simulink library "halout"  (R2021b)
settings: Solver=VariableStepAuto  StartTime=0.0  StopTime=10.0  RelTol=1e-3
undefined symbols (not defined in the file): C_TASK_5MS_S, FALSE, KHAL_CAN1FDAPS3E2E_flg, KHAL_CAN1FDAPS3TxReq_flg, KHAL_CAN1FDVCU2E2E_flg, KHAL_CAN1FDVCU2TxReq_flg, KHAL_CAN1FDVCU3E2E_flg, KHAL_CAN1FDVCU3TxReq_flg, KHAL_CAN1TxReq_flg, KHAL_CAN2TxReq_flg, KHAL_CAN3FDVCU1TxReq_flg, KHAL_CAN3FDVCU2E2E_flg, KHAL_CAN3FDVCU2TxReq_flg, KHAL_CAN3TxReq_flg, KHAL_CAN4FDVCU1E2E_flg, KHAL_CAN4FDVCU1TxReq_flg, KHAL_CAN4TxReq_flg, KHAL_CAN5TxReq_flg, ONE_INT, TRUE, ZERO_INT
libraries: FVT_lib x383, simulink x179
(part 4 of 20)

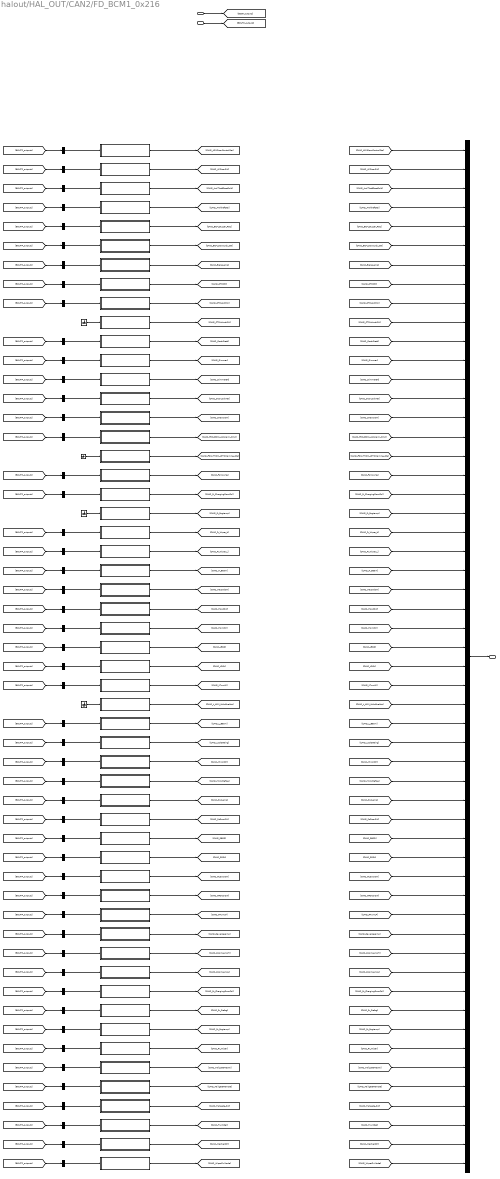
== system halout/HAL_OUT/CAN2/FD_BCM1_0x216 ==
  BSCP_outputs : Inport  OutDataTypeStr=Bus: BSCP_outputs
  BOUTP_outputs : Inport  Port=2  OutDataTypeStr=Bus: BOUTP_outputs
  APMDoorControlSta : Subsystem
  AllDoorSW : Subsystem
  AntiTheftSeatFold : Subsystem
  AntitheftSta : Subsystem
  BCMBuzzerReq : Subsystem
  BCMDoorLockSta : Subsystem
  BrakeLamp : Subsystem
  CTDCtrl : Subsystem
  CTDLockSW : Subsystem
  CTDUnlockSW : Subsystem
  CrashDetd : Subsystem
  Dimmer : Subsystem
  DimmerEN : Subsystem
  DoorLockIND : Subsystem
  DrDoorSW : Subsystem
  FDCBCMLockAlarmCmd : Subsystem
  FDCTHCMAPTCWarningSta : Subsystem
  FollowMe : Subsystem
  FrChargingDoorCtrl : Subsystem
  FrFogLamp : Subsystem
  FrWiperH : Subsystem
  FrWiperL : Subsystem
  Ground{,1..3} (4 alike) : Ground
  HBeam : Subsystem
  HazardSW : Subsystem
  HoodSW : Subsystem
  HornCtrl : Subsystem
  LAPMWdwEnable : Subsystem
  LBSD : Subsystem
  LBeam : Subsystem
  LDRL : Subsystem
  LTurnLP : Subsystem
  LockSetting : Subsystem
  MirrorCtrl : Subsystem
  MirrorDefog : Subsystem
  PosLamp : Subsystem
  PsDoorSW : Subsystem
  RBSD : Subsystem
  RDRL : Subsystem
  RLDoorSW : Subsystem
  RRDoorSW : Subsystem
  RTurnLP : Subsystem
  ReverseLamp : Subsystem
  RoomLampH : Subsystem
  RoomLampL : Subsystem
  RrChargingDoorCtrl : Subsystem
  RrDefog : Subsystem
  RrFogLamp : Subsystem
  RrWiper : Subsystem
  TailgateHDSW : Subsystem
  TailgateRemote : Subsystem
  TailgateSW : Subsystem
  TrunkRel : Subsystem
  WasherCtrl : Subsystem
  WiperFixMode : Subsystem
  bus_creator : BusCreator  Inputs=54  OutDataTypeStr=Bus: DT_CAN2_SG_FD_BCM1  NonVirtualBus=on
  bus_selector : BusSelector  OutputSignals=VOUTP_APMDoorControlSta_flg
  bus_selector1 : BusSelector  OutputSignals=VOUTP_AllDoorSW_flg
  bus_selector10 : BusSelector  OutputSignals=VOUTP_Dimmer_pct
  bus_selector11 : BusSelector  OutputSignals=VOUTP_DimmerEN_flg
  bus_selector12 : BusSelector  OutputSignals=VOUTP_DoorLockIND_flg
  bus_selector13 : BusSelector  OutputSignals=VOUTP_DrDoorSW_flg
  bus_selector14 : BusSelector  OutputSignals=VOUTP_LockAlarm_enum
  bus_selector16 : BusSelector  OutputSignals=VOUTP_FollowMe_flg
  bus_selector17 : BusSelector  OutputSignals=VOUTP_FrChargingDoorCtrl_enum
  bus_selector18 : BusSelector  OutputSignals=VOUTP_FrWiperH_flg
  bus_selector19 : BusSelector  OutputSignals=VOUTP_FrWiperL_flg
  bus_selector2 : BusSelector  OutputSignals=VOUTP_AntitheftSeatFlod_flg
  bus_selector20 : BusSelector  OutputSignals=VOUTP_HBeam_flg
  bus_selector21 : BusSelector  OutputSignals=VOUTP_HazardSW_flg
  bus_selector22 : BusSelector  OutputSignals=VOUTP_HoodSW_flg
  bus_selector23 : BusSelector  OutputSignals=VOUTP_HornCtrl_flg
  bus_selector24 : BusSelector  OutputSignals=VOUTP_LBSD_flg
  bus_selector25 : BusSelector  OutputSignals=VOUTP_LDRL_flg
  bus_selector26 : BusSelector  OutputSignals=VOUTP_LTurnLP_flg
  bus_selector27 : BusSelector  OutputSignals=VOUTP_LBeam_flg
  bus_selector28 : BusSelector  OutputSignals=VOUTP_LockSetting_flg
  bus_selector29 : BusSelector  OutputSignals=VOUTP_MirrorCtrl_enum
  bus_selector3 : BusSelector  OutputSignals=VOUTP_AntitheftSta_enum
  bus_selector30 : BusSelector  OutputSignals=VOUTP_MirrorDefog_flg
  bus_selector31 : BusSelector  OutputSignals=VOUTP_PosLamp_flg
  bus_selector32 : BusSelector  OutputSignals=VOUTP_PsDoorSW_flg
  bus_selector33 : BusSelector  OutputSignals=VOUTP_RBSD_flg
  bus_selector34 : BusSelector  OutputSignals=VOUTP_RDRL_flg
  bus_selector35 : BusSelector  OutputSignals=VOUTP_RLDoorSW_flg
  bus_selector36 : BusSelector  OutputSignals=VOUTP_RRDoorSW_flg
  bus_selector37 : BusSelector  OutputSignals=VOUTP_RTurnLP_flg
  bus_selector38 : BusSelector  OutputSignals=VOUTP_ReverseLamp_flg
  bus_selector39 : BusSelector  OutputSignals=VOUTP_RoomLampH_flg
  bus_selector4 : BusSelector  OutputSignals=VOUTP_BCMBuzzerReq_flg
  bus_selector40 : BusSelector  OutputSignals=VOUTP_RoomLampL_flg
  bus_selector41 : BusSelector  OutputSignals=VOUTP_RrChargingDoorCtrl_enum
  bus_selector42 : BusSelector  OutputSignals=VOUTP_RrDefog_flg
  bus_selector43 : BusSelector  OutputSignals=VOUTP_RrFogLamp_flg
  bus_selector44 : BusSelector  OutputSignals=VOUTP_RrWiper_flg
  bus_selector45 : BusSelector  OutputSignals=VOUTP_TailgateHDSW_flg
  bus_selector46 : BusSelector  OutputSignals=VOUTP_TailgateRemote_enum
  bus_selector47 : BusSelector  OutputSignals=VOUTP_TailgateSW_flg
  bus_selector48 : BusSelector  OutputSignals=VOUTP_TrunkRel_flg
  bus_selector49 : BusSelector  OutputSignals=VOUTP_WasherCtrl_enum
  bus_selector5 : BusSelector  OutputSignals=VOUTP_BCMDoorLockSta_flg
  bus_selector50 : BusSelector  OutputSignals=VOUTP_WiperFixMode_flg
  bus_selector6 : BusSelector  OutputSignals=VOUTP_BrakeLamp_flg
  bus_selector7 : BusSelector  OutputSignals=VOUTP_CTDCtrl_enum
  bus_selector8 : BusSelector  OutputSignals=VOUTP_CTDLockSW_flg
  bus_selector9 : BusSelector  OutputSignals=VOUTP_CrashDetd_flg
  FD_BCM1 : Outport
  wires:
  BSCP_outputs/1 -> [BSCP_outputs]
  BOUTP_outputs/1 -> [BOUTP_outputs]
  [CAN2_APMDoorControlSta] -> bus_creator/1  "CAN2_APMDoorControlSta"
  [CAN2_AllDoorSW] -> bus_creator/2  "CAN2_AllDoorSW"
  [CAN2_AntiTheftSeatFold] -> bus_creator/3  "CAN2_AntiTheftSeatFold"
  [CAN2_AntitheftSta] -> bus_creator/4  "CAN2_AntitheftSta"
  [CAN2_BCM_Buzzer_Req] -> bus_creator/5  "CAN2_BCM_Buzzer_Req"
  [CAN2_BCM_DoorLock_Sta] -> bus_creator/6  "CAN2_BCM_DoorLock_Sta"
  [CAN2_BrakeLamp] -> bus_creator/7  "CAN2_BrakeLamp"
  [CAN2_CTDCtrl] -> bus_creator/8  "CAN2_CTDCtrl"
  [CAN2_CTDLockSW] -> bus_creator/9  "CAN2_CTDLockSW"
  [CAN2_CTDUnlockSW] -> bus_creator/10  "CAN2_CTDUnlockSW"
  [CAN2_CrashDetd] -> bus_creator/11  "CAN2_CrashDetd"
  [CAN2_Dimmer] -> bus_creator/12  "CAN2_Dimmer"
  [CAN2_DimmerEN] -> bus_creator/13  "CAN2_DimmerEN"
  [CAN2_DoorLockIND] -> bus_creator/14  "CAN2_DoorLockIND"
  [CAN2_DrDoorSW] -> bus_creator/15  "CAN2_DrDoorSW"
  [CAN2_FDC_BCM_LockAlarm_Cmd] -> bus_creator/16  "CAN2_FDC_BCM_LockAlarm_Cmd"
  [CAN2_FDC_THCM_APTCWarning_Sta] -> bus_creator/17  "CAN2_FDC_THCM_APTCWarning_Sta"
  [CAN2_FollowMe] -> bus_creator/18  "CAN2_FollowMe"
  [CAN2_Fr_ChargingDoorCtrl] -> bus_creator/19  "CAN2_Fr_ChargingDoorCtrl"
  [CAN2_Fr_FogLamp] -> bus_creator/20  "CAN2_Fr_FogLamp"
  [CAN2_Fr_Wiper_H] -> bus_creator/21  "CAN2_Fr_Wiper_H"
  [CAN2_Fr_Wiper_L] -> bus_creator/22  "CAN2_Fr_Wiper_L"
  [CAN2_H_Beam] -> bus_creator/23  "CAN2_H_Beam"
  [CAN2_HazardSW] -> bus_creator/24  "CAN2_HazardSW"
  [CAN2_HoodSW] -> bus_creator/25  "CAN2_HoodSW"
  [CAN2_HornCtrl] -> bus_creator/26  "CAN2_HornCtrl"
  [CAN2_LBSD] -> bus_creator/27  "CAN2_LBSD"
  [CAN2_LDRL] -> bus_creator/28  "CAN2_LDRL"
  [CAN2_LTurnLP] -> bus_creator/29  "CAN2_LTurnLP"
  [CAN2_L_APM_WdwEnable] -> bus_creator/30  "CAN2_L_APM_WdwEnable"
  [CAN2_L_Beam] -> bus_creator/31  "CAN2_L_Beam"
  [CAN2_LockSetting] -> bus_creator/32  "CAN2_LockSetting"
  [CAN2_MirrorCtrl] -> bus_creator/33  "CAN2_MirrorCtrl"
  [CAN2_MirrorDefog] -> bus_creator/34  "CAN2_MirrorDefog"
  [CAN2_PosLamp] -> bus_creator/35  "CAN2_PosLamp"
  [CAN2_PsDoorSW] -> bus_creator/36  "CAN2_PsDoorSW"
  [CAN2_RBSD] -> bus_creator/37  "CAN2_RBSD"
  [CAN2_RDRL] -> bus_creator/38  "CAN2_RDRL"
  [CAN2_RLDoorSW] -> bus_creator/39  "CAN2_RLDoorSW"
  [CAN2_RRDoorSW] -> bus_creator/40  "CAN2_RRDoorSW"
  [CAN2_RTurnLP] -> bus_creator/41  "CAN2_RTurnLP"
  [CAN2_ReverseLamp] -> bus_creator/42  "CAN2_ReverseLamp"
  [CAN2_RoomLampH] -> bus_creator/43  "CAN2_RoomLampH"
  [CAN2_RoomLampL] -> bus_creator/44  "CAN2_RoomLampL"
  [CAN2_Rr_ChargingDoorCtrl] -> bus_creator/45  "CAN2_Rr_ChargingDoorCtrl"
  [CAN2_Rr_Defog] -> bus_creator/46  "CAN2_Rr_Defog"
  [CAN2_Rr_FogLamp] -> bus_creator/47  "CAN2_Rr_FogLamp"
  [CAN2_Rr_Wiper] -> bus_creator/48  "CAN2_Rr_Wiper"
  [CAN2_TailgateHDSW] -> bus_creator/49  "CAN2_TailgateHDSW"
  [CAN2_TailgateRemote] -> bus_creator/50  "CAN2_TailgateRemote"
  [CAN2_Tailgate_SW] -> bus_creator/51  "CAN2_Tailgate_SW"
  [CAN2_TrunkRel] -> bus_creator/52  "CAN2_TrunkRel"
  [CAN2_WasherCtrl] -> bus_creator/53  "CAN2_WasherCtrl"
  [CAN2_WiperFixMode] -> bus_creator/54  "CAN2_WiperFixMode"
  bus_creator/1 -> FD_BCM1/1
  APMDoorControlSta/1(CAN2_APMDoorControlSta) -> [CAN2_APMDoorControlSta]
  AllDoorSW/1(CAN2_AllDoorSW) -> [CAN2_AllDoorSW]
  AntiTheftSeatFold/1(CAN2_AntiTheftSeatFold) -> [CAN2_AntiTheftSeatFold]
  AntitheftSta/1(CAN2_AntitheftSta) -> [CAN2_AntitheftSta]
  BCMBuzzerReq/1(CAN2_BCM_Buzzer_Req) -> [CAN2_BCM_Buzzer_Req]
  BCMDoorLockSta/1(CAN2_BCM_DoorLock_Sta) -> [CAN2_BCM_DoorLock_Sta]
  BrakeLamp/1(CAN2_BrakeLamp) -> [CAN2_BrakeLamp]
  CTDCtrl/1(CAN2_CTDCtrl) -> [CAN2_CTDCtrl]
  CTDLockSW/1(CAN2_CTDLockSW) -> [CAN2_CTDLockSW]
  CTDUnlockSW/1(CAN2_CTDUnlockSW) -> [CAN2_CTDUnlockSW]
  CrashDetd/1(CAN2_CrashDetd) -> [CAN2_CrashDetd]
  Dimmer/1(CAN2_Dimmer) -> [CAN2_Dimmer]
  DimmerEN/1(CAN2_DimmerEN) -> [CAN2_DimmerEN]
  DoorLockIND/1(CAN2_DoorLockIND) -> [CAN2_DoorLockIND]
  DrDoorSW/1(CAN2_DrDoorSW) -> [CAN2_DrDoorSW]
  FDCBCMLockAlarmCmd/1(CAN2_FDC_BCM_LockAlarm_Cmd) -> [CAN2_FDC_BCM_LockAlarm_Cmd]
  FDCTHCMAPTCWarningSta/1(CAN2_FDC_THCM_APTCWarning_Sta) -> [CAN2_FDC_THCM_APTCWarning_Sta]
  FollowMe/1(CAN2_FollowMe) -> [CAN2_FollowMe]
  FrChargingDoorCtrl/1(CAN2_Fr_ChargingDoorCtrl) -> [CAN2_Fr_ChargingDoorCtrl]
  FrFogLamp/1(CAN2_Fr_FogLamp) -> [CAN2_Fr_FogLamp]
  FrWiperH/1(CAN2_Fr_Wiper_H) -> [CAN2_Fr_Wiper_H]
  FrWiperL/1(CAN2_Fr_Wiper_L) -> [CAN2_Fr_Wiper_L]
  HBeam/1(CAN2_H_Beam) -> [CAN2_H_Beam]
  HazardSW/1(CAN2_HazardSW) -> [CAN2_HazardSW]
  HoodSW/1(CAN2_HoodSW) -> [CAN2_HoodSW]
  HornCtrl/1(CAN2_HornCtrl) -> [CAN2_HornCtrl]
  LBSD/1(CAN2_LBSD) -> [CAN2_LBSD]
  LDRL/1(CAN2_LDRL) -> [CAN2_LDRL]
  LTurnLP/1(CAN2_LTurnLP) -> [CAN2_LTurnLP]
  LAPMWdwEnable/1(CAN2_L_APM_WdwEnable) -> [CAN2_L_APM_WdwEnable]
  LBeam/1(CAN2_L_Beam) -> [CAN2_L_Beam]
  LockSetting/1(CAN2_LockSetting) -> [CAN2_LockSetting]
  MirrorCtrl/1(CAN2_MirrorCtrl) -> [CAN2_MirrorCtrl]
  MirrorDefog/1(CAN2_MirrorDefog) -> [CAN2_MirrorDefog]
  PosLamp/1(CAN2_PosLamp) -> [CAN2_PosLamp]
  PsDoorSW/1(CAN2_PsDoorSW) -> [CAN2_PsDoorSW]
  RBSD/1(CAN2_RBSD) -> [CAN2_RBSD]
  RDRL/1(CAN2_RDRL) -> [CAN2_RDRL]
  RLDoorSW/1(CAN2_RLDoorSW) -> [CAN2_RLDoorSW]
  RRDoorSW/1(CAN2_RRDoorSW) -> [CAN2_RRDoorSW]
  RTurnLP/1(CAN2_RTurnLP) -> [CAN2_RTurnLP]
  ReverseLamp/1(CAN2_ReverseLamp) -> [CAN2_ReverseLamp]
  RoomLampH/1(CAN2_RoomLampH) -> [CAN2_RoomLampH]
  RoomLampL/1(CAN2_RoomLampL) -> [CAN2_RoomLampL]
  RrChargingDoorCtrl/1(CAN2_Rr_ChargingDoorCtrl) -> [CAN2_Rr_ChargingDoorCtrl]
  RrDefog/1(CAN2_Rr_Defog) -> [CAN2_Rr_Defog]
  RrFogLamp/1(CAN2_Rr_FogLamp) -> [CAN2_Rr_FogLamp]
  RrWiper/1(CAN2_Rr_Wiper) -> [CAN2_Rr_Wiper]
  TailgateHDSW/1(CAN2_TailgateHDSW) -> [CAN2_TailgateHDSW]
  TailgateRemote/1(CAN2_TailgateRemote) -> [CAN2_TailgateRemote]
  TailgateSW/1(CAN2_Tailgate_SW) -> [CAN2_Tailgate_SW]
  TrunkRel/1(CAN2_TrunkRel) -> [CAN2_TrunkRel]
  WasherCtrl/1(CAN2_WasherCtrl) -> [CAN2_WasherCtrl]
  WiperFixMode/1(CAN2_WiperFixMode) -> [CAN2_WiperFixMode]
  bus_selector/1 -> APMDoorControlSta/1(APMDoorControlSta)  "<VOUTP_APMDoorControlSta_flg>"
  [BOUTP_outputs] -> bus_selector/1
  bus_selector1/1 -> AllDoorSW/1(AllDoorSW)  "<VOUTP_AllDoorSW_flg>"
  [BOUTP_outputs] -> bus_selector1/1
  bus_selector2/1 -> AntiTheftSeatFold/1(AntiTheftSeatFold)  "<VOUTP_AntitheftSeatFlod_flg>"
  [BOUTP_outputs] -> bus_selector2/1
  bus_selector3/1 -> AntitheftSta/1(AntitheftSta)  "<VOUTP_AntitheftSta_enum>"
  [BOUTP_outputs] -> bus_selector3/1
  bus_selector4/1 -> BCMBuzzerReq/1(BCMBuzzerReq)  "<VOUTP_BCMBuzzerReq_flg>"
  [BOUTP_outputs] -> bus_selector4/1
  bus_selector5/1 -> BCMDoorLockSta/1(BCMDoorLockSta)  "<VOUTP_BCMDoorLockSta_flg>"
  [BOUTP_outputs] -> bus_selector5/1
  bus_selector6/1 -> BrakeLamp/1(BrakeLamp)  "<VOUTP_BrakeLamp_flg>"
  [BOUTP_outputs] -> bus_selector6/1
  bus_selector7/1 -> CTDCtrl/1(CTDCtrl)  "<VOUTP_CTDCtrl_enum>"
  [BOUTP_outputs] -> bus_selector7/1
  bus_selector8/1 -> CTDLockSW/1(CTDLockSW)  "<VOUTP_CTDLockSW_flg>"
  [BOUTP_outputs] -> bus_selector8/1
  Ground/1 -> CTDUnlockSW/1(CTDUnlockSW)
  bus_selector9/1 -> CrashDetd/1(CrashDetd)  "<VOUTP_CrashDetd_flg>"
  [BOUTP_outputs] -> bus_selector9/1
  bus_selector10/1 -> Dimmer/1(Dimmer)  "<VOUTP_Dimmer_pct>"
  [BOUTP_outputs] -> bus_selector10/1
  bus_selector11/1 -> DimmerEN/1(DimmerEN)  "<VOUTP_DimmerEN_flg>"
  [BOUTP_outputs] -> bus_selector11/1
  bus_selector12/1 -> DoorLockIND/1(DoorLockIND)  "<VOUTP_DoorLockIND_flg>"
  [BOUTP_outputs] -> bus_selector12/1
  bus_selector13/1 -> DrDoorSW/1(DrDoorSW)  "<VOUTP_DrDoorSW_flg>"
  [BOUTP_outputs] -> bus_selector13/1
  bus_selector14/1 -> FDCBCMLockAlarmCmd/1(FDCBCMLockAlarmCmd)  "<VOUTP_LockAlarm_enum>"
  [BOUTP_outputs] -> bus_selector14/1
  bus_selector16/1 -> FollowMe/1(FollowMe)  "<VOUTP_FollowMe_flg>"
  [BOUTP_outputs] -> bus_selector16/1
  bus_selector17/1 -> FrChargingDoorCtrl/1(FrChargingDoorCtrl)  "<VOUTP_FrChargingDoorCtrl_enum>"
  [BOUTP_outputs] -> bus_selector17/1
  Ground1/1 -> FrFogLamp/1(FrFogLamp)
  bus_selector18/1 -> FrWiperH/1(FrWiperH)  "<VOUTP_FrWiperH_flg>"
  [BOUTP_outputs] -> bus_selector18/1
  bus_selector19/1 -> FrWiperL/1(FrWiperL)  "<VOUTP_FrWiperL_flg>"
  [BOUTP_outputs] -> bus_selector19/1
  bus_selector20/1 -> HBeam/1(HBeam)  "<VOUTP_HBeam_flg>"
  [BOUTP_outputs] -> bus_selector20/1
  bus_selector21/1 -> HazardSW/1(HazardSW)  "<VOUTP_HazardSW_flg>"
  [BOUTP_outputs] -> bus_selector21/1
  bus_selector22/1 -> HoodSW/1(HoodSW)  "<VOUTP_HoodSW_flg>"
  [BOUTP_outputs] -> bus_selector22/1
  bus_selector23/1 -> HornCtrl/1(HornCtrl)  "<VOUTP_HornCtrl_flg>"
  [BOUTP_outputs] -> bus_selector23/1
  bus_selector24/1 -> LBSD/1(LBSD)  "<VOUTP_LBSD_flg>"
  [BOUTP_outputs] -> bus_selector24/1
  bus_selector25/1 -> LDRL/1(LDRL)  "<VOUTP_LDRL_flg>"
  [BOUTP_outputs] -> bus_selector25/1
  bus_selector26/1 -> LTurnLP/1(LTurnLP)  "<VOUTP_LTurnLP_flg>"
  [BOUTP_outputs] -> bus_selector26/1
  Ground2/1 -> LAPMWdwEnable/1(LAPMWdwEnable)
  bus_selector27/1 -> LBeam/1(LBeam)  "<VOUTP_LBeam_flg>"
  [BOUTP_outputs] -> bus_selector27/1
  bus_selector28/1 -> LockSetting/1(LockSetting)  "<VOUTP_LockSetting_flg>"
  [BOUTP_outputs] -> bus_selector28/1
  bus_selector29/1 -> MirrorCtrl/1(MirrorCtrl)  "<VOUTP_MirrorCtrl_enum>"
  [BOUTP_outputs] -> bus_selector29/1
  bus_selector30/1 -> MirrorDefog/1(MirrorDefog)  "<VOUTP_MirrorDefog_flg>"
  [BOUTP_outputs] -> bus_selector30/1
  bus_selector31/1 -> PosLamp/1(PosLamp)  "<VOUTP_PosLamp_flg>"
  [BOUTP_outputs] -> bus_selector31/1
  bus_selector32/1 -> PsDoorSW/1(PsDoorSW)  "<VOUTP_PsDoorSW_flg>"
  [BOUTP_outputs] -> bus_selector32/1
  bus_selector33/1 -> RBSD/1(RBSD)  "<VOUTP_RBSD_flg>"
  [BOUTP_outputs] -> bus_selector33/1
  bus_selector34/1 -> RDRL/1(RDRL)  "<VOUTP_RDRL_flg>"
  [BOUTP_outputs] -> bus_selector34/1
  bus_selector35/1 -> RLDoorSW/1(RLDoorSW)  "<VOUTP_RLDoorSW_flg>"
  [BOUTP_outputs] -> bus_selector35/1
  bus_selector36/1 -> RRDoorSW/1(RRDoorSW)  "<VOUTP_RRDoorSW_flg>"
  [BOUTP_outputs] -> bus_selector36/1
  bus_selector37/1 -> RTurnLP/1(RTurnLP)  "<VOUTP_RTurnLP_flg>"
  [BOUTP_outputs] -> bus_selector37/1
  bus_selector38/1 -> ReverseLamp/1(ReverseLamp)  "<VOUTP_ReverseLamp_flg>"
  [BOUTP_outputs] -> bus_selector38/1
  bus_selector39/1 -> RoomLampH/1(RoomLampH)  "<VOUTP_RoomLampH_flg>"
  [BOUTP_outputs] -> bus_selector39/1
  bus_selector40/1 -> RoomLampL/1(RoomLampL)  "<VOUTP_RoomLampL_flg>"
  [BOUTP_outputs] -> bus_selector40/1
  bus_selector41/1 -> RrChargingDoorCtrl/1(RrChargingDoorCtrl)  "<VOUTP_RrChargingDoorCtrl_enum>"
  [BOUTP_outputs] -> bus_selector41/1
  bus_selector42/1 -> RrDefog/1(RrDefog)  "<VOUTP_RrDefog_flg>"
  [BOUTP_outputs] -> bus_selector42/1
  bus_selector43/1 -> RrFogLamp/1(RrFogLamp)  "<VOUTP_RrFogLamp_flg>"
  [BOUTP_outputs] -> bus_selector43/1
  bus_selector44/1 -> RrWiper/1(RrWiper)  "<VOUTP_RrWiper_flg>"
  [BOUTP_outputs] -> bus_selector44/1
  bus_selector45/1 -> TailgateHDSW/1(TailgateHDSW)  "<VOUTP_TailgateHDSW_flg>"
  [BOUTP_outputs] -> bus_selector45/1
  bus_selector46/1 -> TailgateRemote/1(TailgateRemote)  "<VOUTP_TailgateRemote_enum>"
  [BOUTP_outputs] -> bus_selector46/1
  bus_selector47/1 -> TailgateSW/1(TailgateSW)  "<VOUTP_TailgateSW_flg>"
  [BOUTP_outputs] -> bus_selector47/1
  bus_selector48/1 -> TrunkRel/1(TrunkRel)  "<VOUTP_TrunkRel_flg>"
  [BOUTP_outputs] -> bus_selector48/1
  bus_selector49/1 -> WasherCtrl/1(WasherCtrl)  "<VOUTP_WasherCtrl_enum>"
  [BOUTP_outputs] -> bus_selector49/1
  bus_selector50/1 -> WiperFixMode/1(WiperFixMode)  "<VOUTP_WiperFixMode_flg>"
  [BOUTP_outputs] -> bus_selector50/1
  Ground3/1 -> FDCTHCMAPTCWarningSta/1(FDCTHCMAPTCWarningSta)

== system halout/HAL_OUT/CAN2/FD_BCM2_0x217 ==
  BSCP_outputs : Inport  OutDataTypeStr=Bus: BSCP_outputs
  BOUTP_outputs : Inport  Port=2  OutDataTypeStr=Bus: BOUTP_outputs
  AmbLightBreath1 : Subsystem
  AmbLightBreath2 : Subsystem
  AmbLightBreath3 : Subsystem
  AmbLightBrightness1 : Subsystem
  AmbLightBrightness2 : Subsystem
  AmbLightBrightness3 : Subsystem
  AmbLightColor1 : Subsystem
  AmbLightColor2 : Subsystem
  AmbLightColor3 : Subsystem
  LampPwr : Subsystem
  User1AmbLightColor : Subsystem
  User1DrAmbLightBrightness : Subsystem
  User1IPAmbLightBrightness : Subsystem
  User2AmbLightColor : Subsystem
  User2DrAmbLightBrightness : Subsystem
  User2IPAmbLightBrightness : Subsystem
  User3AmbLightColor : Subsystem
  User3DrAmbLightBrightness : Subsystem
  User3IPAmbLightBrightness : Subsystem
  User4AmbLightColor : Subsystem
  User4DrAmbLightBrightness : Subsystem
  User4IPAmbLightBrightness : Subsystem
  User5AmbLightColor : Subsystem
  User5DrAmbLightBrightness : Subsystem
  User5IPAmbLightBrightness : Subsystem
  User6AmbLightColor : Subsystem
  User6DrAmbLightBrightness : Subsystem
  User6IPAmbLightBrightness : Subsystem
  bus_creator : BusCreator  Inputs=28  OutDataTypeStr=Bus: DT_CAN2_SG_FD_BCM2  NonVirtualBus=on
  bus_selector : BusSelector  OutputSignals=VOUTP_AmbLightBreath1_flg
  bus_selector1 : BusSelector  OutputSignals=VOUTP_AmbLightBreath2_flg
  bus_selector10 : BusSelector  OutputSignals=VOUTP_User1AmbLightColor_enum
  bus_selector11 : BusSelector  OutputSignals=VOUTP_User1DrAmbLightBrightness_enum
  bus_selector12 : BusSelector  OutputSignals=VOUTP_User1IPAmbLightBrightness_enum
  bus_selector13 : BusSelector  OutputSignals=VOUTP_User2AmbLightColor_enum
  bus_selector14 : BusSelector  OutputSignals=VOUTP_User2DrAmbLightBrightness_enum
  bus_selector15 : BusSelector  OutputSignals=VOUTP_User2IPAmbLightBrightness_enum
  bus_selector16 : BusSelector  OutputSignals=VOUTP_User3AmbLightColor_enum
  bus_selector17 : BusSelector  OutputSignals=VOUTP_User3DrAmbLightBrightness_enum
  bus_selector18 : BusSelector  OutputSignals=VOUTP_User3IPAmbLightBrightness_enum
  bus_selector19 : BusSelector  OutputSignals=VOUTP_User4AmbLightColor_enum
  bus_selector2 : BusSelector  OutputSignals=VOUTP_AmbLightBreath3_flg
  bus_selector20 : BusSelector  OutputSignals=VOUTP_User4DrAmbLightBrightness_enum
  bus_selector21 : BusSelector  OutputSignals=VOUTP_User4IPAmbLightBrightness_enum
  bus_selector22 : BusSelector  OutputSignals=VOUTP_User5AmbLightColor_enum
  bus_selector23 : BusSelector  OutputSignals=VOUTP_User5DrAmbLightBrightness_enum
  bus_selector24 : BusSelector  OutputSignals=VOUTP_User5IPAmbLightBrightness_enum
  bus_selector25 : BusSelector  OutputSignals=VOUTP_User6AmbLightColor_enum
  bus_selector26 : BusSelector  OutputSignals=VOUTP_User6DrAmbLightBrightness_enum
  bus_selector27 : BusSelector  OutputSignals=VOUTP_User6IPAmbLightBrightness_enum
  bus_selector3 : BusSelector  OutputSignals=VOUTP_AmbLightBrightness1_enum
  bus_selector4 : BusSelector  OutputSignals=VOUTP_AmbLightBrightness2_enum
  bus_selector5 : BusSelector  OutputSignals=VOUTP_AmbLightBrightness3_enum
  bus_selector6 : BusSelector  OutputSignals=VOUTP_AmbLightColor1_enum
  bus_selector7 : BusSelector  OutputSignals=VOUTP_AmbLightColor2_enum
  bus_selector8 : BusSelector  OutputSignals=VOUTP_AmbLightColor3_enum
  bus_selector9 : BusSelector  OutputSignals=VOUTP_LampPwr_flg
  FD_BCM2 : Outport
  wires:
  BSCP_outputs/1 -> [BSCP_outputs]
  BOUTP_outputs/1 -> [BOUTP_outputs]
  [CAN2_AmbLightBreath1] -> bus_creator/1  "CAN2_AmbLightBreath1"
  [CAN2_AmbLightBreath2] -> bus_creator/2  "CAN2_AmbLightBreath2"
  [CAN2_AmbLightBreath3] -> bus_creator/3  "CAN2_AmbLightBreath3"
  [CAN2_AmbLightBrightness1] -> bus_creator/4  "CAN2_AmbLightBrightness1"
  [CAN2_AmbLightBrightness2] -> bus_creator/5  "CAN2_AmbLightBrightness2"
  [CAN2_AmbLightBrightness3] -> bus_creator/6  "CAN2_AmbLightBrightness3"
  [CAN2_AmbLightColor1] -> bus_creator/7  "CAN2_AmbLightColor1"
  [CAN2_AmbLightColor2] -> bus_creator/8  "CAN2_AmbLightColor2"
  [CAN2_AmbLightColor3] -> bus_creator/9  "CAN2_AmbLightColor3"
  [CAN2_LampPwr] -> bus_creator/10  "CAN2_LampPwr"
  [CAN2_User1AmbLightColor] -> bus_creator/11  "CAN2_User1AmbLightColor"
  [CAN2_User1DrAmbLightBrightness] -> bus_creator/12  "CAN2_User1DrAmbLightBrightness"
  [CAN2_User1IPAmbLightBrightness] -> bus_creator/13  "CAN2_User1IPAmbLightBrightness"
  [CAN2_User2AmbLightColor] -> bus_creator/14  "CAN2_User2AmbLightColor"
  [CAN2_User2DrAmbLightBrightness] -> bus_creator/15  "CAN2_User2DrAmbLightBrightness"
  [CAN2_User2IPAmbLightBrightness] -> bus_creator/16  "CAN2_User2IPAmbLightBrightness"
  [CAN2_User3AmbLightColor] -> bus_creator/17  "CAN2_User3AmbLightColor"
  [CAN2_User3DrAmbLightBrightness] -> bus_creator/18  "CAN2_User3DrAmbLightBrightness"
  [CAN2_User3IPAmbLightBrightness] -> bus_creator/19  "CAN2_User3IPAmbLightBrightness"
  [CAN2_User4AmbLightColor] -> bus_creator/20  "CAN2_User4AmbLightColor"
  [CAN2_User4DrAmbLightBrightness] -> bus_creator/21  "CAN2_User4DrAmbLightBrightness"
  [CAN2_User4IPAmbLightBrightness] -> bus_creator/22  "CAN2_User4IPAmbLightBrightness"
  [CAN2_User5AmbLightColor] -> bus_creator/23  "CAN2_User5AmbLightColor"
  [CAN2_User5DrAmbLightBrightness] -> bus_creator/24  "CAN2_User5DrAmbLightBrightness"
  [CAN2_User5IPAmbLightBrightness] -> bus_creator/25  "CAN2_User5IPAmbLightBrightness"
  [CAN2_User6AmbLightColor] -> bus_creator/26  "CAN2_User6AmbLightColor"
  [CAN2_User6DrAmbLightBrightness] -> bus_creator/27  "CAN2_User6DrAmbLightBrightness"
  [CAN2_User6IPAmbLightBrightness] -> bus_creator/28  "CAN2_User6IPAmbLightBrightness"
  bus_creator/1 -> FD_BCM2/1
  AmbLightBreath1/1(CAN2_AmbLightBreath1) -> [CAN2_AmbLightBreath1]
  AmbLightBreath2/1(CAN2_AmbLightBreath2) -> [CAN2_AmbLightBreath2]
  AmbLightBreath3/1(CAN2_AmbLightBreath3) -> [CAN2_AmbLightBreath3]
  AmbLightBrightness1/1(CAN2_AmbLightBrightness1) -> [CAN2_AmbLightBrightness1]
  AmbLightBrightness2/1(CAN2_AmbLightBrightness2) -> [CAN2_AmbLightBrightness2]
  AmbLightBrightness3/1(CAN2_AmbLightBrightness3) -> [CAN2_AmbLightBrightness3]
  AmbLightColor1/1(CAN2_AmbLightColor1) -> [CAN2_AmbLightColor1]
  AmbLightColor2/1(CAN2_AmbLightColor2) -> [CAN2_AmbLightColor2]
  AmbLightColor3/1(CAN2_AmbLightColor3) -> [CAN2_AmbLightColor3]
  LampPwr/1(CAN2_LampPwr) -> [CAN2_LampPwr]
  User1AmbLightColor/1(CAN2_User1AmbLightColor) -> [CAN2_User1AmbLightColor]
  User1DrAmbLightBrightness/1(CAN2_User1DrAmbLightBrightness) -> [CAN2_User1DrAmbLightBrightness]
  User1IPAmbLightBrightness/1(CAN2_User1IPAmbLightBrightness) -> [CAN2_User1IPAmbLightBrightness]
  User2AmbLightColor/1(CAN2_User2AmbLightColor) -> [CAN2_User2AmbLightColor]
  User2DrAmbLightBrightness/1(CAN2_User2DrAmbLightBrightness) -> [CAN2_User2DrAmbLightBrightness]
  User2IPAmbLightBrightness/1(CAN2_User2IPAmbLightBrightness) -> [CAN2_User2IPAmbLightBrightness]
  User3AmbLightColor/1(CAN2_User3AmbLightColor) -> [CAN2_User3AmbLightColor]
  User3DrAmbLightBrightness/1(CAN2_User3DrAmbLightBrightness) -> [CAN2_User3DrAmbLightBrightness]
  User3IPAmbLightBrightness/1(CAN2_User3IPAmbLightBrightness) -> [CAN2_User3IPAmbLightBrightness]
  User4AmbLightColor/1(CAN2_User4AmbLightColor) -> [CAN2_User4AmbLightColor]
  User4DrAmbLightBrightness/1(CAN2_User4DrAmbLightBrightness) -> [CAN2_User4DrAmbLightBrightness]
  User4IPAmbLightBrightness/1(CAN2_User4IPAmbLightBrightness) -> [CAN2_User4IPAmbLightBrightness]
  User5AmbLightColor/1(CAN2_User5AmbLightColor) -> [CAN2_User5AmbLightColor]
  User5DrAmbLightBrightness/1(CAN2_User5DrAmbLightBrightness) -> [CAN2_User5DrAmbLightBrightness]
  User5IPAmbLightBrightness/1(CAN2_User5IPAmbLightBrightness) -> [CAN2_User5IPAmbLightBrightness]
  User6AmbLightColor/1(CAN2_User6AmbLightColor) -> [CAN2_User6AmbLightColor]
  User6DrAmbLightBrightness/1(CAN2_User6DrAmbLightBrightness) -> [CAN2_User6DrAmbLightBrightness]
  User6IPAmbLightBrightness/1(CAN2_User6IPAmbLightBrightness) -> [CAN2_User6IPAmbLightBrightness]
  bus_selector/1 -> AmbLightBreath1/1(AmbLightBreath1)  "<VOUTP_AmbLightBreath1_flg>"
  [BOUTP_outputs] -> bus_selector/1
  bus_selector1/1 -> AmbLightBreath2/1(AmbLightBreath2)  "<VOUTP_AmbLightBreath2_flg>"
  [BOUTP_outputs] -> bus_selector1/1
  bus_selector2/1 -> AmbLightBreath3/1(AmbLightBreath3)  "<VOUTP_AmbLightBreath3_flg>"
  [BOUTP_outputs] -> bus_selector2/1
  bus_selector3/1 -> AmbLightBrightness1/1(AmbLightBrightness1)  "<VOUTP_AmbLightBrightness1_enum>"
  [BOUTP_outputs] -> bus_selector3/1
  bus_selector4/1 -> AmbLightBrightness2/1(AmbLightBrightness2)  "<VOUTP_AmbLightBrightness2_enum>"
  [BOUTP_outputs] -> bus_selector4/1
  bus_selector5/1 -> AmbLightBrightness3/1(AmbLightBrightness3)  "<VOUTP_AmbLightBrightness3_enum>"
  [BOUTP_outputs] -> bus_selector5/1
  bus_selector6/1 -> AmbLightColor1/1(AmbLightColor1)  "<VOUTP_AmbLightColor1_enum>"
  [BOUTP_outputs] -> bus_selector6/1
  bus_selector7/1 -> AmbLightColor2/1(AmbLightColor2)  "<VOUTP_AmbLightColor2_enum>"
  [BOUTP_outputs] -> bus_selector7/1
  bus_selector8/1 -> AmbLightColor3/1(AmbLightColor3)  "<VOUTP_AmbLightColor3_enum>"
  [BOUTP_outputs] -> bus_selector8/1
  bus_selector9/1 -> LampPwr/1(LampPwr)  "<VOUTP_LampPwr_flg>"
  [BOUTP_outputs] -> bus_selector9/1
  bus_selector10/1 -> User1AmbLightColor/1(User1AmbLightColor)  "<VOUTP_User1AmbLightColor_enum>"
  [BOUTP_outputs] -> bus_selector10/1
  bus_selector11/1 -> User1DrAmbLightBrightness/1(User1DrAmbLightBrightness)  "<VOUTP_User1DrAmbLightBrightness_enum>"
  [BOUTP_outputs] -> bus_selector11/1
  bus_selector12/1 -> User1IPAmbLightBrightness/1(User1IPAmbLightBrightness)  "<VOUTP_User1IPAmbLightBrightness_enum>"
  [BOUTP_outputs] -> bus_selector12/1
  bus_selector13/1 -> User2AmbLightColor/1(User2AmbLightColor)  "<VOUTP_User2AmbLightColor_enum>"
  [BOUTP_outputs] -> bus_selector13/1
  bus_selector14/1 -> User2DrAmbLightBrightness/1(User2DrAmbLightBrightness)  "<VOUTP_User2DrAmbLightBrightness_enum>"
  [BOUTP_outputs] -> bus_selector14/1
  bus_selector15/1 -> User2IPAmbLightBrightness/1(User2IPAmbLightBrightness)  "<VOUTP_User2IPAmbLightBrightness_enum>"
  [BOUTP_outputs] -> bus_selector15/1
  bus_selector16/1 -> User3AmbLightColor/1(User3AmbLightColor)  "<VOUTP_User3AmbLightColor_enum>"
  [BOUTP_outputs] -> bus_selector16/1
  bus_selector17/1 -> User3DrAmbLightBrightness/1(User3DrAmbLightBrightness)  "<VOUTP_User3DrAmbLightBrightness_enum>"
  [BOUTP_outputs] -> bus_selector17/1
  bus_selector18/1 -> User3IPAmbLightBrightness/1(User3IPAmbLightBrightness)  "<VOUTP_User3IPAmbLightBrightness_enum>"
  [BOUTP_outputs] -> bus_selector18/1
  bus_selector19/1 -> User4AmbLightColor/1(User4AmbLightColor)  "<VOUTP_User4AmbLightColor_enum>"
  [BOUTP_outputs] -> bus_selector19/1
  bus_selector20/1 -> User4DrAmbLightBrightness/1(User4DrAmbLightBrightness)  "<VOUTP_User4DrAmbLightBrightness_enum>"
  [BOUTP_outputs] -> bus_selector20/1
  bus_selector21/1 -> User4IPAmbLightBrightness/1(User4IPAmbLightBrightness)  "<VOUTP_User4IPAmbLightBrightness_enum>"
  [BOUTP_outputs] -> bus_selector21/1
  bus_selector22/1 -> User5AmbLightColor/1(User5AmbLightColor)  "<VOUTP_User5AmbLightColor_enum>"
  [BOUTP_outputs] -> bus_selector22/1
  bus_selector23/1 -> User5DrAmbLightBrightness/1(User5DrAmbLightBrightness)  "<VOUTP_User5DrAmbLightBrightness_enum>"
  [BOUTP_outputs] -> bus_selector23/1
  bus_selector24/1 -> User5IPAmbLightBrightness/1(User5IPAmbLightBrightness)  "<VOUTP_User5IPAmbLightBrightness_enum>"
  [BOUTP_outputs] -> bus_selector24/1
  bus_selector25/1 -> User6AmbLightColor/1(User6AmbLightColor)  "<VOUTP_User6AmbLightColor_enum>"
  [BOUTP_outputs] -> bus_selector25/1
  bus_selector26/1 -> User6DrAmbLightBrightness/1(User6DrAmbLightBrightness)  "<VOUTP_User6DrAmbLightBrightness_enum>"
  [BOUTP_outputs] -> bus_selector26/1
  bus_selector27/1 -> User6IPAmbLightBrightness/1(User6IPAmbLightBrightness)  "<VOUTP_User6IPAmbLightBrightness_enum>"
  [BOUTP_outputs] -> bus_selector27/1

== system halout/HAL_OUT/CAN2/FD_THCM1_0x182 ==
  BSCP_outputs : Inport  OutDataTypeStr=Bus: BSCP_outputs
  BOUTP_outputs : Inport  Port=2  OutDataTypeStr=Bus: BOUTP_outputs
  BatteryMode : Subsystem
  CCUACLampSts : Subsystem
  CCUACMaxLampSts : Subsystem
  CCUAutoLampSts : Subsystem
  CCUAutoMidLampSts : Subsystem
  CCUDispalyRequest : Subsystem
  CCUEcoSts : Subsystem
  CCUFrtOnOffLampSts : Subsystem
  CCUHEATMaxLampSts : Subsystem
  CCURrOnOffLampSts : Subsystem
  CCUSyncLampSts : Subsystem
  CabinMode : Subsystem
  EDriveMode : Subsystem
  FDAGSCmd : Subsystem
  FDRecyAutoCmd : Subsystem
  FrCoolantflow : Subsystem
  FrCoolanttemp : Subsystem
  Ground{,1..17} (18 alike) : Ground
  HPThermalRecoveryReq : Subsystem
  RrCoolantflow : Subsystem
  RrCoolanttemp : Subsystem
  bus_creator : BusCreator  Inputs=37  OutDataTypeStr=Bus: DT_CAN2_SG_FD_THCM1  NonVirtualBus=on
  bus_selector : BusSelector  OutputSignals=VOUTP_BatteryMode_enum
  bus_selector1 : BusSelector  OutputSignals=VOUTP_CCUACLampSts_flg
  bus_selector10 : BusSelector  OutputSignals=VOUTP_sigAmbAirT_C
  bus_selector11 : BusSelector  OutputSignals=VOUTP_sigCbnAirT_C
  bus_selector12 : BusSelector  OutputSignals=VOUTP_sigCbnSolarLeft_W
  bus_selector13 : BusSelector  OutputSignals=VOUTP_sigCbnSolarRight_W
  bus_selector14 : BusSelector  OutputSignals=VOUTP_sigClntTHvBattOut_C
  bus_selector15 : BusSelector  OutputSignals=VOUTP_sigRecircSt_flg
  bus_selector16 : BusSelector  OutputSignals=VOUTP_sigSetTempZon1St_C
  bus_selector17 : BusSelector  OutputSignals=VOUTP_sigSetTempZon2St_C
  bus_selector18 : BusSelector  OutputSignals=VOUTP_sigWindDirZon1St_enum
  bus_selector2 : BusSelector  OutputSignals=VOUTP_CCUACMaxLampSts_flg
  bus_selector3 : BusSelector  OutputSignals=VOUTP_CCUAutoLampSts_flg
  bus_selector4 : BusSelector  OutputSignals=VOUTP_CCUSyncLampSts_flg
  bus_selector5 : BusSelector  OutputSignals=VOUTP_CabinMode_enum
  bus_selector6 : BusSelector  OutputSignals=VOUTP_EDriveMode_enum
  bus_selector7 : BusSelector  OutputSignals=VOUTP_FDAGSCmd_enum
  bus_selector8 : BusSelector  OutputSignals=VOUTP_FDRecyAutoCmd_enum
  bus_selector9 : BusSelector  OutputSignals=VOUTP_sigAirIntenZon1St_enum
  sigAirIntenZon1St : Subsystem
  sigAirIntenZon3St : Subsystem
  sigAmbAirT : Subsystem
  sigCbnAirT : Subsystem
  sigCbnPTCPwrAct : Subsystem
  sigCbnSolarLeft : Subsystem
  sigCbnSolarRight : Subsystem
  sigClmtCmprPwrAct : Subsystem
  sigClntTHvBattOut : Subsystem
  sigDfrstSt : Subsystem
  sigHvacSt : Subsystem
  sigRecircSt : Subsystem
  sigSetTempZon1St : Subsystem
  sigSetTempZon2St : Subsystem
  sigSetTempZon3St : Subsystem
  sigWindDirZon1St : Subsystem
  sigWindDirZon3St : Subsystem
  FD_THCM1 : Outport
  wires:
  BSCP_outputs/1 -> [BSCP_outputs]
  BOUTP_outputs/1 -> [BOUTP_outputs]
  [CAN2_BatteryMode] -> bus_creator/1  "CAN2_BatteryMode"
  [CAN2_CCU_ACLampSts] -> bus_creator/2  "CAN2_CCU_ACLampSts"
  [CAN2_CCU_ACMaxLampSts] -> bus_creator/3  "CAN2_CCU_ACMaxLampSts"
  [CAN2_CCU_AutoLampSts] -> bus_creator/4  "CAN2_CCU_AutoLampSts"
  [CAN2_CCU_AutoMidLampSts] -> bus_creator/5  "CAN2_CCU_AutoMidLampSts"
  [CAN2_CCU_Dispaly_Request] -> bus_creator/6  "CAN2_CCU_Dispaly_Request"
  [CAN2_CCU_EcoSts] -> bus_creator/7  "CAN2_CCU_EcoSts"
  [CAN2_CCU_FrtOnOffLampSts] -> bus_creator/8  "CAN2_CCU_FrtOnOffLampSts"
  [CAN2_CCU_HEATMaxLampSts] -> bus_creator/9  "CAN2_CCU_HEATMaxLampSts"
  [CAN2_CCU_RrOnOffLampSts] -> bus_creator/10  "CAN2_CCU_RrOnOffLampSts"
  [CAN2_CCU_SyncLampSts] -> bus_creator/11  "CAN2_CCU_SyncLampSts"
  [CAN2_CabinMode] -> bus_creator/12  "CAN2_CabinMode"
  [CAN2_EDriveMode] -> bus_creator/13  "CAN2_EDriveMode"
  [CAN2_FD_AGS_Cmd] -> bus_creator/14  "CAN2_FD_AGS_Cmd"
  [CAN2_FD_RecyAuto_Cmd] -> bus_creator/15  "CAN2_FD_RecyAuto_Cmd"
  [CAN2_Fr_Coolantflow] -> bus_creator/16  "CAN2_Fr_Coolantflow"
  [CAN2_Fr_Coolanttemp] -> bus_creator/17  "CAN2_Fr_Coolanttemp"
  [CAN2_HPThermalRecoveryReq] -> bus_creator/18  "CAN2_HPThermalRecoveryReq"
  [CAN2_Rr_Coolantflow] -> bus_creator/19  "CAN2_Rr_Coolantflow"
  [CAN2_Rr_Coolanttemp] -> bus_creator/20  "CAN2_Rr_Coolanttemp"
  [CAN2_sigAirIntenZon1St] -> bus_creator/21  "CAN2_sigAirIntenZon1St"
  [CAN2_sigAirIntenZon3St] -> bus_creator/22  "CAN2_sigAirIntenZon3St"
  [CAN2_sigAmbAirT] -> bus_creator/23  "CAN2_sigAmbAirT"
  [CAN2_sigCbnAirT] -> bus_creator/24  "CAN2_sigCbnAirT"
  [CAN2_sigCbnPTCPwrAct] -> bus_creator/25  "CAN2_sigCbnPTCPwrAct"
  [CAN2_sigCbnSolarLeft] -> bus_creator/26  "CAN2_sigCbnSolarLeft"
  [CAN2_sigCbnSolarRight] -> bus_creator/27  "CAN2_sigCbnSolarRight"
  [CAN2_sigClmtCmprPwrAct] -> bus_creator/28  "CAN2_sigClmtCmprPwrAct"
  [CAN2_sigClntTHvBattOut] -> bus_creator/29  "CAN2_sigClntTHvBattOut"
  [CAN2_sigDfrstSt] -> bus_creator/30  "CAN2_sigDfrstSt"
  [CAN2_sigHvacSt] -> bus_creator/31  "CAN2_sigHvacSt"
  [CAN2_sigRecircSt] -> bus_creator/32  "CAN2_sigRecircSt"
  [CAN2_sigSetTempZon1St] -> bus_creator/33  "CAN2_sigSetTempZon1St"
  [CAN2_sigSetTempZon2St] -> bus_creator/34  "CAN2_sigSetTempZon2St"
  [CAN2_sigSetTempZon3St] -> bus_creator/35  "CAN2_sigSetTempZon3St"
  [CAN2_sigWindDirZon1St] -> bus_creator/36  "CAN2_sigWindDirZon1St"
  [CAN2_sigWindDirZon3St] -> bus_creator/37  "CAN2_sigWindDirZon3St"
  bus_creator/1 -> FD_THCM1/1
  BatteryMode/1(CAN2_BatteryMode) -> [CAN2_BatteryMode]
  CCUACLampSts/1(CAN2_CCU_ACLampSts) -> [CAN2_CCU_ACLampSts]
  CCUACMaxLampSts/1(CAN2_CCU_ACMaxLampSts) -> [CAN2_CCU_ACMaxLampSts]
  CCUAutoLampSts/1(CAN2_CCU_AutoLampSts) -> [CAN2_CCU_AutoLampSts]
  CCUAutoMidLampSts/1(CAN2_CCU_AutoMidLampSts) -> [CAN2_CCU_AutoMidLampSts]
  CCUDispalyRequest/1(CAN2_CCU_Dispaly_Request) -> [CAN2_CCU_Dispaly_Request]
  CCUEcoSts/1(CAN2_CCU_EcoSts) -> [CAN2_CCU_EcoSts]
  CCUFrtOnOffLampSts/1(CAN2_CCU_FrtOnOffLampSts) -> [CAN2_CCU_FrtOnOffLampSts]
  CCUHEATMaxLampSts/1(CAN2_CCU_HEATMaxLampSts) -> [CAN2_CCU_HEATMaxLampSts]
  CCURrOnOffLampSts/1(CAN2_CCU_RrOnOffLampSts) -> [CAN2_CCU_RrOnOffLampSts]
  CCUSyncLampSts/1(CAN2_CCU_SyncLampSts) -> [CAN2_CCU_SyncLampSts]
  CabinMode/1(CAN2_CabinMode) -> [CAN2_CabinMode]
  EDriveMode/1(CAN2_EDriveMode) -> [CAN2_EDriveMode]
  FDAGSCmd/1(CAN2_FD_AGS_Cmd) -> [CAN2_FD_AGS_Cmd]
  FDRecyAutoCmd/1(CAN2_FD_RecyAuto_Cmd) -> [CAN2_FD_RecyAuto_Cmd]
  FrCoolantflow/1(CAN2_Fr_Coolantflow) -> [CAN2_Fr_Coolantflow]
  FrCoolanttemp/1(CAN2_Fr_Coolanttemp) -> [CAN2_Fr_Coolanttemp]
  HPThermalRecoveryReq/1(CAN2_HPThermalRecoveryReq) -> [CAN2_HPThermalRecoveryReq]
  RrCoolantflow/1(CAN2_Rr_Coolantflow) -> [CAN2_Rr_Coolantflow]
  RrCoolanttemp/1(CAN2_Rr_Coolanttemp) -> [CAN2_Rr_Coolanttemp]
  sigAirIntenZon1St/1(CAN2_sigAirIntenZon1St) -> [CAN2_sigAirIntenZon1St]
  sigAirIntenZon3St/1(CAN2_sigAirIntenZon3St) -> [CAN2_sigAirIntenZon3St]
  sigAmbAirT/1(CAN2_sigAmbAirT) -> [CAN2_sigAmbAirT]
  sigCbnAirT/1(CAN2_sigCbnAirT) -> [CAN2_sigCbnAirT]
  sigCbnPTCPwrAct/1(CAN2_sigCbnPTCPwrAct) -> [CAN2_sigCbnPTCPwrAct]
  sigCbnSolarLeft/1(CAN2_sigCbnSolarLeft) -> [CAN2_sigCbnSolarLeft]
  sigCbnSolarRight/1(CAN2_sigCbnSolarRight) -> [CAN2_sigCbnSolarRight]
  sigClmtCmprPwrAct/1(CAN2_sigClmtCmprPwrAct) -> [CAN2_sigClmtCmprPwrAct]
  sigClntTHvBattOut/1(CAN2_sigClntTHvBattOut) -> [CAN2_sigClntTHvBattOut]
  sigDfrstSt/1(CAN2_sigDfrstSt) -> [CAN2_sigDfrstSt]
  sigHvacSt/1(CAN2_sigHvacSt) -> [CAN2_sigHvacSt]
  sigRecircSt/1(CAN2_sigRecircSt) -> [CAN2_sigRecircSt]
  sigSetTempZon1St/1(CAN2_sigSetTempZon1St) -> [CAN2_sigSetTempZon1St]
  sigSetTempZon2St/1(CAN2_sigSetTempZon2St) -> [CAN2_sigSetTempZon2St]
  sigSetTempZon3St/1(CAN2_sigSetTempZon3St) -> [CAN2_sigSetTempZon3St]
  sigWindDirZon1St/1(CAN2_sigWindDirZon1St) -> [CAN2_sigWindDirZon1St]
  sigWindDirZon3St/1(CAN2_sigWindDirZon3St) -> [CAN2_sigWindDirZon3St]
  bus_selector/1 -> BatteryMode/1(BatteryMode)  "<VOUTP_BatteryMode_enum>"
  [BOUTP_outputs] -> bus_selector/1
  bus_selector1/1 -> CCUACLampSts/1(CCUACLampSts)  "<VOUTP_CCUACLampSts_flg>"
  [BOUTP_outputs] -> bus_selector1/1
  bus_selector2/1 -> CCUACMaxLampSts/1(CCUACMaxLampSts)  "<VOUTP_CCUACMaxLampSts_flg>"
  [BOUTP_outputs] -> bus_selector2/1
  bus_selector3/1 -> CCUAutoLampSts/1(CCUAutoLampSts)  "<VOUTP_CCUAutoLampSts_flg>"
  [BOUTP_outputs] -> bus_selector3/1
  Ground/1 -> CCUAutoMidLampSts/1(CCUAutoMidLampSts)
  Ground1/1 -> CCUDispalyRequest/1(CCUDispalyRequest)
  Ground2/1 -> CCUEcoSts/1(CCUEcoSts)
  Ground3/1 -> CCUFrtOnOffLampSts/1(CCUFrtOnOffLampSts)
  Ground4/1 -> CCUHEATMaxLampSts/1(CCUHEATMaxLampSts)
  Ground5/1 -> CCURrOnOffLampSts/1(CCURrOnOffLampSts)
  bus_selector4/1 -> CCUSyncLampSts/1(CCUSyncLampSts)  "<VOUTP_CCUSyncLampSts_flg>"
  [BOUTP_outputs] -> bus_selector4/1
  bus_selector5/1 -> CabinMode/1(CabinMode)  "<VOUTP_CabinMode_enum>"
  [BOUTP_outputs] -> bus_selector5/1
  bus_selector6/1 -> EDriveMode/1(EDriveMode)  "<VOUTP_EDriveMode_enum>"
  [BOUTP_outputs] -> bus_selector6/1
  bus_selector7/1 -> FDAGSCmd/1(FDAGSCmd)  "<VOUTP_FDAGSCmd_enum>"
  [BOUTP_outputs] -> bus_selector7/1
  bus_selector8/1 -> FDRecyAutoCmd/1(FDRecyAutoCmd)  "<VOUTP_FDRecyAutoCmd_enum>"
  [BOUTP_outputs] -> bus_selector8/1
  Ground6/1 -> FrCoolantflow/1(FrCoolantflow)
  Ground7/1 -> FrCoolanttemp/1(FrCoolanttemp)
  Ground8/1 -> HPThermalRecoveryReq/1(HPThermalRecoveryReq)
  Ground9/1 -> RrCoolantflow/1(RrCoolantflow)
  Ground10/1 -> RrCoolanttemp/1(RrCoolanttemp)
  bus_selector9/1 -> sigAirIntenZon1St/1(sigAirIntenZon1St)  "<VOUTP_sigAirIntenZon1St_enum>"
  [BOUTP_outputs] -> bus_selector9/1
  Ground11/1 -> sigAirIntenZon3St/1(sigAirIntenZon3St)
  bus_selector10/1 -> sigAmbAirT/1(sigAmbAirT)  "<VOUTP_sigAmbAirT_C>"
  [BOUTP_outputs] -> bus_selector10/1
  bus_selector11/1 -> sigCbnAirT/1(sigCbnAirT)  "<VOUTP_sigCbnAirT_C>"
  [BOUTP_outputs] -> bus_selector11/1
  Ground12/1 -> sigCbnPTCPwrAct/1(sigCbnPTCPwrAct)
  bus_selector12/1 -> sigCbnSolarLeft/1(sigCbnSolarLeft)  "<VOUTP_sigCbnSolarLeft_W>"
  [BOUTP_outputs] -> bus_selector12/1
  bus_selector13/1 -> sigCbnSolarRight/1(sigCbnSolarRight)  "<VOUTP_sigCbnSolarRight_W>"
  [BOUTP_outputs] -> bus_selector13/1
  Ground13/1 -> sigClmtCmprPwrAct/1(sigClmtCmprPwrAct)
  bus_selector14/1 -> sigClntTHvBattOut/1(sigClntTHvBattOut)  "<VOUTP_sigClntTHvBattOut_C>"
  [BOUTP_outputs] -> bus_selector14/1
  Ground14/1 -> sigDfrstSt/1(sigDfrstSt)
  Ground15/1 -> sigHvacSt/1(sigHvacSt)
  bus_selector15/1 -> sigRecircSt/1(sigRecircSt)  "<VOUTP_sigRecircSt_flg>"
  [BOUTP_outputs] -> bus_selector15/1
  bus_selector16/1 -> sigSetTempZon1St/1(sigSetTempZon1St)  "<VOUTP_sigSetTempZon1St_C>"
  [BOUTP_outputs] -> bus_selector16/1
  bus_selector17/1 -> sigSetTempZon2St/1(sigSetTempZon2St)  "<VOUTP_sigSetTempZon2St_C>"
  [BOUTP_outputs] -> bus_selector17/1
  Ground16/1 -> sigSetTempZon3St/1(sigSetTempZon3St)
  bus_selector18/1 -> sigWindDirZon1St/1(sigWindDirZon1St)  "<VOUTP_sigWindDirZon1St_enum>"
  [BOUTP_outputs] -> bus_selector18/1
  Ground17/1 -> sigWindDirZon3St/1(sigWindDirZon3St)
